simulink model "crank_cam_generator_2017b"  (R2017b)
settings: Solver=FixedStepDiscrete  StartTime=0.0  StopTime=10.0  FixedStep=1e-4  RelTol=1e-3
InitFcn:
  | mbd_pnt_consistency_checks(bdroot(gcs));
undefined symbols (not defined in the file): B14, C10, G7, M16
libraries: mbd_pnt_ec_toolbox x4, simulink x1
settings Model: Creator=sgulgonul  LastModifiedBy=oolonthegreat
settings DataIOCC: ExternalInput=off  InitialState=off  SaveOutput=off  SignalLogging=off  SaveTime=off
settings OptimizationCC: DefaultParameterBehavior=Inlined  EnhancedBackFolding=on  PassReuseOutputArgsAs=Individual arguments  OptimizeBlockOrder=speed  DifferentSizesBufferReuse=on
settings DebuggingCC: InheritedTsInSrcMsg=none  SingleTaskRateTransMsg=error  ParameterTunabilityLossMsg=error  UnconnectedInputMsg=error  UnconnectedOutputMsg=error  UnconnectedLineMsg=error  UnknownTsInhSupMsg=error
settings HardwareCC: ProdBitPerPointer=32  ProdBitPerSizeT=32  ProdBitPerPtrDiffT=32  ProdLargestAtomicInteger=Long  ProdLargestAtomicFloat=Double  ProdEndianess=BigEndian  ProdWordSize=32  ProdHWDeviceType=Motorola PowerPC
settings SFSimCC: MATLABDynamicMemAlloc=off
settings RTWCC: SystemTargetFile=mbd_pnt.tlc  MakeCommand=mbd_pnt_make_rtw COPY_MDLREF_INCLUDES=0  TemplateMakefile=mbd_pnt.tmf  PostCodeGenCommand=mbd_pnt_analyzegencode(buildInfo)  Description=Model Based Design Toolbox MPC574xP Code Generation Target  GenerateReport=on  IncludeHyperlinkInReport=on  LaunchReport=on  GenerateTraceInfo=on  GenerateTraceReport=on  GenerateTraceReportSl=on  GenerateTraceReportSf=on  GenerateTraceReportEml=on
settings CodeAppCC: ForceParamTrailComments=on  IgnoreCustomStorageClasses=off  OperatorAnnotations=on  SimulinkDataObjDesc=on  SFDataObjDesc=on  InsertBlockDesc=on
settings STFCustomTargetCC: TargetLangStandard=C99 (ISO)  MultiwordLength=256  CombineOutputUpdateFcns=on  SuppressErrorStatus=on  ERTCustomFileBanners=on  SupportContinuousTime=off  SupportNonInlinedSFcns=off  RemoveResetFunc=on  MATLABClassNameForMDSCustomization=Simulink.SoftwareTarget.ERTCustomization  GRTInterface=off  SystemTargetFile=mbd_pnt.tlc
settings ERTTargetCC: TargetLangStandard=C99 (ISO)  ParMdlRefBuildCompliant=off  CompOptLevelCompliant=off  ConcurrentExecutionCompliant=off  SuppressErrorStatus=on  ModelStepFunctionPrototypeControlCompliant=off  CPPClassGenCompliant=off  UseToolchainInfoCompliant=off  InlinedParameterPlacement=NonHierarchical  ERTCustomFileTemplate=example_file_process.tlc

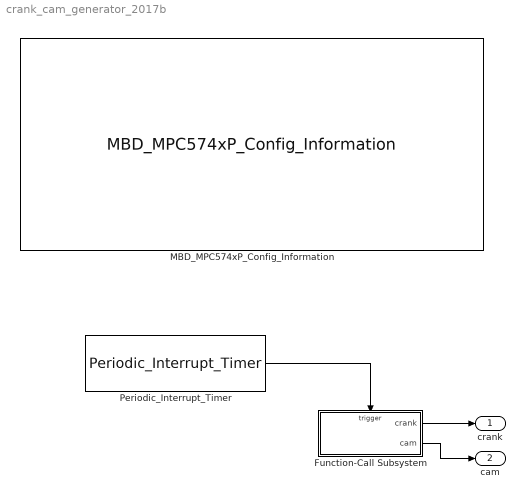
== system crank_cam_generator_2017b ==
  Function-Call Subsystem : Subsystem  TreatAsAtomicUnit=on
  MBD_MPC574xP_Config_Information : mbd_pnt_ec_toolbox/MPC574xP/MBD_MPC574xP_Config_Information  disp_str=|  config_params=[]
      | System Clock : 200 MHz
      | Target : MPC5744P
      | Package : 144LQFP
      | XTAL Freq : 40 MHz
      | Compiler : S32 Design Studio
      | Target Type : SRAM
      | Global Interrupt Priority : 8
      | System Tick Interrupt Priority : 12
      | Freemaster : Serial1 (115200 Kbits)
      | Download Code after build : (COM5,115200)
      settings: SourceProductName=Model Based Design Toolbox for MPC574xP
  Periodic_Interrupt_Timer : mbd_pnt_ec_toolbox/MPC574xP/Utility Blocks/Periodic_Interrupt_Timer  pit_chan=1  pit_timeout=0.4  int_priority=15  pit_timeout_val=19999
      settings: SourceProductName=Model Based Design Toolbox for MPC574xP
  crank : Outport
  cam : Outport  Port=2
  wires:
  Periodic_Interrupt_Timer/1 -> Function-Call Subsystem/Trigger
  Function-Call Subsystem/2(cam) -> cam/1
  Function-Call Subsystem/1(crank) -> crank/1

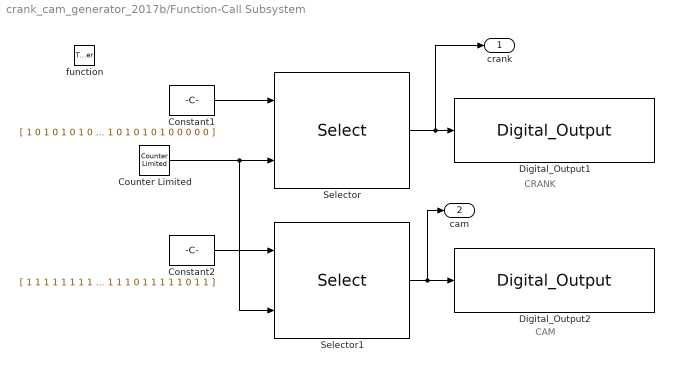
== system crank_cam_generator_2017b/Function-Call Subsystem ==
  note: CRANK
  note: CAM
  function : TriggerPort  TriggerType=function-call  VariantControl=Variant
  Constant1 : Constant  Value=[ 1 0 1 0 1 0 1 0 1 0 1 0 1 0 1 0 1 0 1 0 1 0 1 0 1 0 1 0 1 0 1 0 1 0 1 0 0 0 0 0 1 0 1 0 1 0 1 0 1 0 1 0 1 0 1 0 1 0 1 0 1 0 1 0 1 0 1 0 1 0 1 0 1 0 1 0 0 0 0 0 1 0 1 0 1 0 1 0 1 0 1 0 1 0 1 0 1 0 1 0 1 0 1 0 1 0 1 0 1 0 1 0 1 0 1 0 0 0 0 0 1 0 1 0 1 0 1 0 1 0 1 0 1 0 1 0 1 0 1 0 1 0 1 0 1 0 1 0 1 0 1 0 1 0 1 0 0 0 0 0 1 0 1 0 1 0 1 0 1 0 1 0 1 0 1 0 1 0 1 0 1 0 1 0 1 0 1 0 1 0 1 0 1 0 1 0 0 0 0 0 1 0 1 0 1 0 1 0 1 0 1 0 1 0 1 0 1 0 1 0 1 0 1 0 1 0 1 0 1 0 1 0 1 0 1 0 0 0 0 0 ]  OutDataTypeStr=boolean
  Constant2 : Constant  Value=[ 1 1 1 1 1 1 1 1 1 1 1 1 1 1 1 1 1 1 1 1 1 1 1 1 1 1 1 1 1 1 1 1 1 1 1 1 1 0 1 1 1 1 1 1 1 1 1 1 1 1 1 1 1 1 1 1 1 1 1 1 1 1 1 1 1 1 1 1 1 1 1 1 1 1 1 1 1 0 1 1 1 1 1 1 1 1 1 1 1 1 1 1 1 1 1 1 1 1 1 1 1 1 1 1 1 1 1 1 1 1 1 1 1 1 1 1 1 0 1 1 1 1 1 1 1 1 1 1 1 1 1 1 1 1 1 1 1 1 1 1 1 1 1 1 1 1 1 1 1 1 1 1 1 1 1 1 1 0 1 1 1 1 1 1 1 1 1 1 1 1 1 1 1 1 1 1 1 1 1 1 1 1 1 1 1 1 1 1 1 1 1 1 1 1 1 1 1 0 1 1 1 1 1 1 1 1 1 1 1 1 1 1 1 1 1 1 1 1 1 1 1 1 1 1 1 1 1 1 1 1 1 0 1 1 1 1 1 0 1 1 ]  OutDataTypeStr=boolean
  Counter Limited : simulink/Sources/Counter Limited  uplimit=239  tsamp=-1
  Digital_Output1 : mbd_pnt_ec_toolbox/MPC574xP/Peripheral Interface Blocks/Digital_Output  gpio_outputs="42   : C10 :  [111] : [136] : [B14]"  pinNum=[111]  pcrNum=42
      settings: SourceProductName=Model Based Design Toolbox for MPC574xP
  Digital_Output2 : mbd_pnt_ec_toolbox/MPC574xP/Peripheral Interface Blocks/Digital_Output  gpio_outputs="103 : G7   :  [83]   : [104] : [M16]"  pinNum=[83]  pcrNum=103
      settings: SourceProductName=Model Based Design Toolbox for MPC574xP
  Selector : Selector  IndexMode=Zero-based  InputPortWidth=240  IndexOptions=Index vector (port)  Indices=[1 3]  OutputSizes=1
  Selector1 : Selector  IndexMode=Zero-based  InputPortWidth=240  IndexOptions=Index vector (port)  Indices=[1 3]  OutputSizes=1
  crank : Outport
  cam : Outport  Port=2
  wires:
  Selector1/1 -> cam/1, Digital_Output2/1
  Selector/1 -> crank/1, Digital_Output1/1
  Constant1/1 -> Selector/1
  Counter Limited/1 -> Selector1/2, Selector/2
  Constant2/1 -> Selector1/1
